simulink model "simulink_group46"  (R2022b)
settings: Solver=FixedStepAuto  StartTime=0.0  StopTime=10  FixedStep=1e-3  RelTol=1e-3  EnableMultiTasking=on
undefined symbols (not defined in the file): A0, A1, D0, D1, D10, D11, D12, D13, D2, D3, D4, D5, D6, D7, D8, D9, PTA0, PTA1, PTA2, PTB2, PTB23, PTB3, PTB9, PTC16, PTC17, PTC2, PTC3, PTC4, PTD0, PTD1, PTD2, PTD3
libraries: frdmk64flib x20, etargetslib x18, simulink x2, dspstat3 x1
(part 2 of 2)

== stateflow chart simulink_group46/Requirements Table ==
  (default) -> (junction 1073756783)
  (junction 1073756783) -> (junction 1073756784) : {
      | % SF_REQ_REV_07
      | }
  (junction 1073756784) -> (junction 1073756786) : {
      | % HEADER_ASSIGNMENTS
      |
      | }
  (junction 1073756786) -> (junction 1073756788) : {
      | % START_A_4
      | }
  (junction 1073756788) -> (junction 1073756790) : {
      | }
  (junction 1073756790) -> (junction 1073756792) : {
      | reqtable_assumption((LRL <= 175 && LRL >= 30 && LRL <= URL), 4);
      | }
  (junction 1073756792) -> (junction 1073756794) : {
      | }
  (junction 1073756794) -> (junction 1073756796) : {
      | % END_A_4
      | }
  (junction 1073756796) -> (junction 1073756798) : {
      | % START_A_7
      | }
  (junction 1073756798) -> (junction 1073756800) : {
      | }
  (junction 1073756800) -> (junction 1073756802) : {
      | reqtable_assumption((URL <= 175 && URL >= 50), 7);
      | }
  (junction 1073756802) -> (junction 1073756804) : {
      | }
  (junction 1073756804) -> (junction 1073756806) : {
      | % END_A_7
      | }
  (junction 1073756806) -> (junction 1073756808) : {
      | % START_A_10
      | }
  (junction 1073756808) -> (junction 1073756810) : {
      | }
  (junction 1073756810) -> (junction 1073756812) : {
      | reqtable_assumption((PACING_REF_PWM <= 64), 10);
      | }
  (junction 1073756812) -> (junction 1073756814) : {
      | }
  (junction 1073756814) -> (junction 1073756816) : {
      | % END_A_10
      | }
  (junction 1073756816) -> (junction 1073756818) : {
      | % START_A_16
      | }
  (junction 1073756818) -> (junction 1073756820) : {
      | }
  (junction 1073756820) -> (junction 1073756822) : {
      | reqtable_assumption((VRP >= 150 && VRP <= 500), 16);
      | }
  (junction 1073756822) -> (junction 1073756824) : {
      | }
  (junction 1073756824) -> (junction 1073756826) : {
      | % END_A_16
      | }
  (junction 1073756826) -> (junction 1073756828) : {
      | % START_A_19
      | }
  (junction 1073756828) -> (junction 1073756830) : {
      | }
  (junction 1073756830) -> (junction 1073756832) : {
      | reqtable_assumption((ARP >= 150 && ARP <= 500), 19);
      | }
  (junction 1073756832) -> (junction 1073756834) : {
      | }
  (junction 1073756834) -> (junction 1073756836) : {
      | % END_A_19
      | }
  (junction 1073756836) -> (junction 1073756838) : {
      | % START_A_22
      | }
  (junction 1073756838) -> (junction 1073756840) : {
      | }
  (junction 1073756840) -> (junction 1073756842) : {
      | reqtable_assumption((mode >= 0 && mode <= 8), 22);
      | }
  (junction 1073756842) -> (junction 1073756844) : {
      | }
  (junction 1073756844) -> (junction 1073756846) : {
      | % END_A_22
      | }
  (junction 1073756846) -> (junction 1073756848) : {
      | % START_R_1
      | }
  (junction 1073756848) -> (junction 1073756850) : {
      | }
  (junction 1073756850) -> (junction 1073756852)
  (junction 1073756852) -> (junction 1073756854) [order 1] : [(((mode) == (2))) && (((FRONTEND_CTRL) == (true))) && (((PACE_CHARGE_CTRL) == (true))) && (((PACE_GND_CTRL) == (true))) && (((ATR_CMP_DETECT) == (true)) || ((ATR_CMP_DETECT) == (false)))]
  (junction 1073756852) -> (junction 1073756896) [order 2]
  (junction 1073756854) -> (junction 1073756856) : {
      | reqtable_postcondition((((ATR_PACE_CTRL) == (false))) && (((ATR_GND_CTRL) == (true)) || ((ATR_GND_CTRL) == (false))), 'R:1');
      |
      |
      | }
  (junction 1073756856) -> (junction 1073756858) : {
      | }
  (junction 1073756858) -> (junction 1073756860) : {
      | % START_R_79
      | }
  (junction 1073756860) -> (junction 1073756862) : {
      | }
  (junction 1073756862) -> (junction 1073756864)
  (junction 1073756864) -> (junction 1073756866) [order 1] : [(((VENT_CMP_DETECT) == (false))) && (((prev_state) == (2)))]
  (junction 1073756864) -> (junction 1073756872) [order 2]
  (junction 1073756866) -> (junction 1073756868) : {
      | reqtable_postcondition((((VENT_PACE_CTRL) == (true))) && (((VENT_GND_CTRL) == (true))) && (((state) == (3))), 'R:1.1');
      |
      |
      | }
  (junction 1073756868) -> (junction 1073756870) : {
      | }
  (junction 1073756870) -> (junction 1073756872)
  (junction 1073756872) -> (junction 1073756874)
  (junction 1073756874) -> (junction 1073756876) : {
      | % END_R_79
      | }
  (junction 1073756876) -> (junction 1073756878) : {
      | % START_R_82
      | }
  (junction 1073756878) -> (junction 1073756880) : {
      | }
  (junction 1073756880) -> (junction 1073756882)
  (junction 1073756882) -> (junction 1073756884) [order 1] : [(((VENT_CMP_DETECT) == (true))) && (((prev_state) == (1)))]
  (junction 1073756882) -> (junction 1073756890) [order 2]
  (junction 1073756884) -> (junction 1073756886) : {
      | reqtable_postcondition((((VENT_PACE_CTRL) == (false))) && (((VENT_GND_CTRL) == (false))) && (((state) == (1))), 'R:1.2');
      |
      |
      | }
  (junction 1073756886) -> (junction 1073756888) : {
      | }
  (junction 1073756888) -> (junction 1073756890)
  (junction 1073756890) -> (junction 1073756892)
  (junction 1073756892) -> (junction 1073756894) : {
      | % END_R_82
      | }
  (junction 1073756894) -> (junction 1073756896)
  (junction 1073756896) -> (junction 1073756898)
  (junction 1073756898) -> (junction 1073756900) : {
      | % END_R_1
      | }
  (junction 1073756900) -> (junction 1073756902) : {
      | % START_R_28
      | }
  (junction 1073756902) -> (junction 1073756904) : {
      | }
  (junction 1073756904) -> (junction 1073756906)
  (junction 1073756906) -> (junction 1073756908) [order 1] : [(((mode) == (1)) || ((mode) == (2))) && (((FRONTEND_CTRL) == (false))) && (((PACE_CHARGE_CTRL) == (false))) && (((PACE_GND_CTRL) == (true))) && (((VENT_CMP_DETECT) == (false))) && (((ATR_CMP_DETECT) == (true)) || ((ATR_CMP_DETECT) == (false))) && (((prev_state) == (1)))]
  (junction 1073756906) -> (junction 1073756914) [order 2]
  (junction 1073756908) -> (junction 1073756910) : {
      | reqtable_postcondition((((VENT_PACE_CTRL) == (true))) && (((ATR_PACE_CTRL) == (false))) && (((VENT_GND_CTRL) == (false))) && (((ATR_GND_CTRL) == (true)) || ((ATR_GND_CTRL) == (false))) && (((state) == (1))), 'R:2');
      |
      |
      | }
  (junction 1073756910) -> (junction 1073756912) : {
      | }
  (junction 1073756912) -> (junction 1073756914)
  (junction 1073756914) -> (junction 1073756916)
  (junction 1073756916) -> (junction 1073756918) : {
      | % END_R_28
      | }
  (junction 1073756918) -> (junction 1073756920) : {
      | % START_R_46
      | }
  (junction 1073756920) -> (junction 1073756922) : {
      | }
  (junction 1073756922) -> (junction 1073756924) : {
      |
      |
      | }
  (junction 1073756924) -> (junction 1073756926) : {
      | }
  (junction 1073756926) -> (junction 1073756928) : {
      | % START_R_61
      | }
  (junction 1073756928) -> (junction 1073756930) : {
      | }
  (junction 1073756930) -> (junction 1073756932)
  (junction 1073756932) -> (junction 1073756934) [order 1] : [(((mode) == (1))) && (((FRONTEND_CTRL) == (false))) && (((PACE_CHARGE_CTRL) == (true))) && (((PACE_GND_CTRL) == (true))) && (((VENT_CMP_DETECT) == (true)) || ((VENT_CMP_DETECT) == (false))) && (((ATR_CMP_DETECT) == (true)) || ((ATR_CMP_DETECT) == (false))) && (((prev_state) == (2)))]
  (junction 1073756932) -> (junction 1073756940) [order 2]
  (junction 1073756934) -> (junction 1073756936) : {
      | reqtable_postcondition((((VENT_PACE_CTRL) == (false))) && (((ATR_PACE_CTRL) == (true)) || ((ATR_PACE_CTRL) == (false))) && (((VENT_GND_CTRL) == (true))) && (((ATR_GND_CTRL) == (true)) || ((ATR_GND_CTRL) == (false))) && (((state) == (2))), 'R:3.1');
      |
      |
      | }
  (junction 1073756936) -> (junction 1073756938) : {
      | }
  (junction 1073756938) -> (junction 1073756940)
  (junction 1073756940) -> (junction 1073756942)
  (junction 1073756942) -> (junction 1073756944) : {
      | % END_R_61
      | }
  (junction 1073756944) -> (junction 1073756946) : {
      | % START_R_64
      | }
  (junction 1073756946) -> (junction 1073756948) : {
      | }
  (junction 1073756948) -> (junction 1073756950)
  (junction 1073756950) -> (junction 1073756952) [order 1] : [(((mode) == (2))) && (((FRONTEND_CTRL) == (true)) || ((FRONTEND_CTRL) == (false))) && (((PACE_CHARGE_CTRL) == (true))) && (((PACE_GND_CTRL) == (true))) && (((VENT_CMP_DETECT) == (true)) || ((VENT_CMP_DETECT) == (false))) && (((ATR_CMP_DETECT) == (true)) || ((ATR_CMP_DETECT) == (false))) && (((prev_state) == (1)))]
  (junction 1073756950) -> (junction 1073756958) [order 2]
  (junction 1073756952) -> (junction 1073756954) : {
      | reqtable_postcondition((((VENT_PACE_CTRL) == (false))) && (((ATR_PACE_CTRL) == (true)) || ((ATR_PACE_CTRL) == (false))) && (((VENT_GND_CTRL) == (true))) && (((ATR_GND_CTRL) == (true)) || ((ATR_GND_CTRL) == (false))) && (((state) == (2))), 'R:3.2');
      |
      |
      | }
  (junction 1073756954) -> (junction 1073756956) : {
      | }
  (junction 1073756956) -> (junction 1073756958)
  (junction 1073756958) -> (junction 1073756960)
  (junction 1073756960) -> (junction 1073756962) : {
      | % END_R_64
      | }
  (junction 1073756962) -> (junction 1073756964) : {
      | % END_R_46
      | }
  (junction 1073756964) -> (junction 1073756966) : {
      | % START_R_31
      | }
  (junction 1073756966) -> (junction 1073756968) : {
      | }
  (junction 1073756968) -> (junction 1073756970)
  (junction 1073756970) -> (junction 1073756972) [order 1] : [(((mode) == (4))) && (((FRONTEND_CTRL) == (true))) && (((PACE_CHARGE_CTRL) == (true))) && (((PACE_GND_CTRL) == (true))) && (((VENT_CMP_DETECT) == (true)) || ((VENT_CMP_DETECT) == (false)))]
  (junction 1073756970) -> (junction 1073757014) [order 2]
  (junction 1073756972) -> (junction 1073756974) : {
      | reqtable_postcondition((((VENT_PACE_CTRL) == (false))) && (((VENT_GND_CTRL) == (true)) || ((VENT_GND_CTRL) == (false))), 'R:4');
      |
      |
      | }
  (junction 1073756974) -> (junction 1073756976) : {
      | }
  (junction 1073756976) -> (junction 1073756978) : {
      | % START_R_85
      | }
  (junction 1073756978) -> (junction 1073756980) : {
      | }
  (junction 1073756980) -> (junction 1073756982)
  (junction 1073756982) -> (junction 1073756984) [order 1] : [(((ATR_CMP_DETECT) == (false))) && (((prev_state) == (2)))]
  (junction 1073756982) -> (junction 1073756990) [order 2]
  (junction 1073756984) -> (junction 1073756986) : {
      | reqtable_postcondition((((ATR_PACE_CTRL) == (true))) && (((ATR_GND_CTRL) == (true))) && (((state) == (3))), 'R:4.1');
      |
      |
      | }
  (junction 1073756986) -> (junction 1073756988) : {
      | }
  (junction 1073756988) -> (junction 1073756990)
  (junction 1073756990) -> (junction 1073756992)
  (junction 1073756992) -> (junction 1073756994) : {
      | % END_R_85
      | }
  (junction 1073756994) -> (junction 1073756996) : {
      | % START_R_88
      | }
  (junction 1073756996) -> (junction 1073756998) : {
      | }
  (junction 1073756998) -> (junction 1073757000)
  (junction 1073757000) -> (junction 1073757002) [order 1] : [(((ATR_CMP_DETECT) == (true))) && (((prev_state) == (1)))]
  (junction 1073757000) -> (junction 1073757008) [order 2]
  (junction 1073757002) -> (junction 1073757004) : {
      | reqtable_postcondition((((ATR_PACE_CTRL) == (false))) && (((ATR_GND_CTRL) == (false))) && (((state) == (1))), 'R:4.2');
      |
      |
      | }
  (junction 1073757004) -> (junction 1073757006) : {
      | }
  (junction 1073757006) -> (junction 1073757008)
  (junction 1073757008) -> (junction 1073757010)
  (junction 1073757010) -> (junction 1073757012) : {
      | % END_R_88
      | }
  (junction 1073757012) -> (junction 1073757014)
  (junction 1073757014) -> (junction 1073757016)
  (junction 1073757016) -> (junction 1073757018) : {
      | % END_R_31
      | }
  (junction 1073757018) -> (junction 1073757020) : {
      | % START_R_37
      | }
  (junction 1073757020) -> (junction 1073757022) : {
      | }
  (junction 1073757022) -> (junction 1073757024)
  (junction 1073757024) -> (junction 1073757026) [order 1] : [(((mode) == (3)) || ((mode) == (4))) && (((FRONTEND_CTRL) == (false))) && (((PACE_CHARGE_CTRL) == (false))) && (((PACE_GND_CTRL) == (true))) && (((VENT_CMP_DETECT) == (true)) || ((VENT_CMP_DETECT) == (false))) && (((ATR_CMP_DETECT) == (false))) && (((prev_state) == (1)))]
  (junction 1073757024) -> (junction 1073757032) [order 2]
  (junction 1073757026) -> (junction 1073757028) : {
      | reqtable_postcondition((((VENT_PACE_CTRL) == (false))) && (((ATR_PACE_CTRL) == (true))) && (((VENT_GND_CTRL) == (true)) || ((VENT_GND_CTRL) == (false))) && (((ATR_GND_CTRL) == (false))) && (((state) == (1))), 'R:5');
      |
      |
      | }
  (junction 1073757028) -> (junction 1073757030) : {
      | }
  (junction 1073757030) -> (junction 1073757032)
  (junction 1073757032) -> (junction 1073757034)
  (junction 1073757034) -> (junction 1073757036) : {
      | % END_R_37
      | }
  (junction 1073757036) -> (junction 1073757038) : {
      | % START_R_55
      | }
  (junction 1073757038) -> (junction 1073757040) : {
      | }
  (junction 1073757040) -> (junction 1073757042) : {
      |
      |
      | }
  (junction 1073757042) -> (junction 1073757044) : {
      | }
  (junction 1073757044) -> (junction 1073757046) : {
      | % START_R_67
      | }
  (junction 1073757046) -> (junction 1073757048) : {
      | }
  (junction 1073757048) -> (junction 1073757050)
  (junction 1073757050) -> (junction 1073757052) [order 1] : [(((mode) == (3))) && (((FRONTEND_CTRL) == (false))) && (((PACE_CHARGE_CTRL) == (true))) && (((PACE_GND_CTRL) == (true))) && (((VENT_CMP_DETECT) == (true)) || ((VENT_CMP_DETECT) == (false))) && (((ATR_CMP_DETECT) == (true)) || ((ATR_CMP_DETECT) == (false))) && (((prev_state) == (2)))]
  (junction 1073757050) -> (junction 1073757058) [order 2]
  (junction 1073757052) -> (junction 1073757054) : {
      | reqtable_postcondition((((VENT_PACE_CTRL) == (true)) || ((VENT_PACE_CTRL) == (false))) && (((ATR_PACE_CTRL) == (false))) && (((VENT_GND_CTRL) == (true)) || ((VENT_GND_CTRL) == (false))) && (((ATR_GND_CTRL) == (true))) && (((state) == (2))), 'R:6.1');
      |
      |
      | }
  (junction 1073757054) -> (junction 1073757056) : {
      | }
  (junction 1073757056) -> (junction 1073757058)
  (junction 1073757058) -> (junction 1073757060)
  (junction 1073757060) -> (junction 1073757062) : {
      | % END_R_67
      | }
  (junction 1073757062) -> (junction 1073757064) : {
      | % START_R_70
      | }
  (junction 1073757064) -> (junction 1073757066) : {
      | }
  (junction 1073757066) -> (junction 1073757068)
  (junction 1073757068) -> (junction 1073757070) [order 1] : [(((mode) == (4))) && (((FRONTEND_CTRL) == (true)) || ((FRONTEND_CTRL) == (false))) && (((PACE_CHARGE_CTRL) == (true))) && (((PACE_GND_CTRL) == (true))) && (((VENT_CMP_DETECT) == (true)) || ((VENT_CMP_DETECT) == (false))) && (((ATR_CMP_DETECT) == (true)) || ((ATR_CMP_DETECT) == (false))) && (((prev_state) == (1)))]
  (junction 1073757068) -> (junction 1073757076) [order 2]
  (junction 1073757070) -> (junction 1073757072) : {
      | reqtable_postcondition((((VENT_PACE_CTRL) == (true)) || ((VENT_PACE_CTRL) == (false))) && (((ATR_PACE_CTRL) == (false))) && (((VENT_GND_CTRL) == (true)) || ((VENT_GND_CTRL) == (false))) && (((ATR_GND_CTRL) == (true))) && (((state) == (2))), 'R:6.2');
      |
      |
      | }
  (junction 1073757072) -> (junction 1073757074) : {
      | }
  (junction 1073757074) -> (junction 1073757076)
  (junction 1073757076) -> (junction 1073757078)
  (junction 1073757078) -> (junction 1073757080) : {
      | % END_R_70
      | }
  (junction 1073757080) -> (junction 1073757082) : {
      | % END_R_55
      | }
  (junction 1073757082) -> (junction 1073757084) : {
      | % START_R_91
      | }
  (junction 1073757084) -> (junction 1073757086) : {
      | }
  (junction 1073757086) -> (junction 1073757088)
  (junction 1073757088) -> (junction 1073757090) [order 1] : [(((mode) == (6))) && (((FRONTEND_CTRL) == (true))) && (((PACE_CHARGE_CTRL) == (true))) && (((PACE_GND_CTRL) == (true))) && (((ATR_CMP_DETECT) == (true)) || ((ATR_CMP_DETECT) == (false)))]
  (junction 1073757088) -> (junction 1073757132) [order 2]
  (junction 1073757090) -> (junction 1073757092) : {
      | reqtable_postcondition((((ATR_PACE_CTRL) == (false))) && (((ATR_GND_CTRL) == (true)) || ((ATR_GND_CTRL) == (false))), 'R:7');
      |
      |
      | }
  (junction 1073757092) -> (junction 1073757094) : {
      | }
  (junction 1073757094) -> (junction 1073757096) : {
      | % START_R_94
      | }
  (junction 1073757096) -> (junction 1073757098) : {
      | }
  (junction 1073757098) -> (junction 1073757100)
  (junction 1073757100) -> (junction 1073757102) [order 1] : [(((VENT_CMP_DETECT) == (false))) && (((prev_state) == (2)))]
  (junction 1073757100) -> (junction 1073757108) [order 2]
  (junction 1073757102) -> (junction 1073757104) : {
      | reqtable_postcondition((((VENT_PACE_CTRL) == (true))) && (((VENT_GND_CTRL) == (true))) && (((state) == (3))), 'R:7.1');
      |
      |
      | }
  (junction 1073757104) -> (junction 1073757106) : {
      | }
  (junction 1073757106) -> (junction 1073757108)
  (junction 1073757108) -> (junction 1073757110)
  (junction 1073757110) -> (junction 1073757112) : {
      | % END_R_94
      | }
  (junction 1073757112) -> (junction 1073757114) : {
      | % START_R_97
      | }
  (junction 1073757114) -> (junction 1073757116) : {
      | }
  (junction 1073757116) -> (junction 1073757118)
  (junction 1073757118) -> (junction 1073757120) [order 1] : [(((VENT_CMP_DETECT) == (true))) && (((prev_state) == (1)))]
  (junction 1073757118) -> (junction 1073757126) [order 2]
  (junction 1073757120) -> (junction 1073757122) : {
      | reqtable_postcondition((((VENT_PACE_CTRL) == (false))) && (((VENT_GND_CTRL) == (false))) && (((state) == (1))), 'R:7.2');
      |
      |
      | }
  (junction 1073757122) -> (junction 1073757124) : {
      | }
  (junction 1073757124) -> (junction 1073757126)
  (junction 1073757126) -> (junction 1073757128)
  (junction 1073757128) -> (junction 1073757130) : {
      | % END_R_97
      | }
  (junction 1073757130) -> (junction 1073757132)
  (junction 1073757132) -> (junction 1073757134)
  (junction 1073757134) -> (junction 1073757136) : {
      | % END_R_91
      | }
  (junction 1073757136) -> (junction 1073757138) : {
      | % START_R_100
      | }
  (junction 1073757138) -> (junction 1073757140) : {
      | }
  (junction 1073757140) -> (junction 1073757142)
  (junction 1073757142) -> (junction 1073757144) [order 1] : [(((mode) == (5)) || ((mode) == (6))) && (((FRONTEND_CTRL) == (false))) && (((PACE_CHARGE_CTRL) == (false))) && (((PACE_GND_CTRL) == (true))) && (((VENT_CMP_DETECT) == (false))) && (((ATR_CMP_DETECT) == (true)) || ((ATR_CMP_DETECT) == (false))) && (((prev_state) == (1)))]
  (junction 1073757142) -> (junction 1073757150) [order 2]
  (junction 1073757144) -> (junction 1073757146) : {
      | reqtable_postcondition((((VENT_PACE_CTRL) == (true))) && (((ATR_PACE_CTRL) == (false))) && (((VENT_GND_CTRL) == (false))) && (((ATR_GND_CTRL) == (true)) || ((ATR_GND_CTRL) == (false))) && (((state) == (1))), 'R:8');
      |
      |
      | }
  (junction 1073757146) -> (junction 1073757148) : {
      | }
  (junction 1073757148) -> (junction 1073757150)
  (junction 1073757150) -> (junction 1073757152)
  (junction 1073757152) -> (junction 1073757154) : {
      | % END_R_100
      | }
  (junction 1073757154) -> (junction 1073757156) : {
      | % START_R_103
      | }
  (junction 1073757156) -> (junction 1073757158) : {
      | }
  (junction 1073757158) -> (junction 1073757160) : {
      |
      |
      | }
  (junction 1073757160) -> (junction 1073757162) : {
      | }
  (junction 1073757162) -> (junction 1073757164) : {
      | % START_R_106
      | }
  (junction 1073757164) -> (junction 1073757166) : {
      | }
  (junction 1073757166) -> (junction 1073757168)
  (junction 1073757168) -> (junction 1073757170) [order 1] : [(((mode) == (5))) && (((FRONTEND_CTRL) == (false))) && (((PACE_CHARGE_CTRL) == (true))) && (((PACE_GND_CTRL) == (true))) && (((VENT_CMP_DETECT) == (true)) || ((VENT_CMP_DETECT) == (false))) && (((ATR_CMP_DETECT) == (true)) || ((ATR_CMP_DETECT) == (false))) && (((prev_state) == (2)))]
  (junction 1073757168) -> (junction 1073757176) [order 2]
  (junction 1073757170) -> (junction 1073757172) : {
      | reqtable_postcondition((((VENT_PACE_CTRL) == (false))) && (((ATR_PACE_CTRL) == (true)) || ((ATR_PACE_CTRL) == (false))) && (((VENT_GND_CTRL) == (true))) && (((ATR_GND_CTRL) == (true)) || ((ATR_GND_CTRL) == (false))) && (((state) == (2))), 'R:9.1');
      |
      |
      | }
  (junction 1073757172) -> (junction 1073757174) : {
      | }
  (junction 1073757174) -> (junction 1073757176)
  (junction 1073757176) -> (junction 1073757178)
  (junction 1073757178) -> (junction 1073757180) : {
      | % END_R_106
      | }
  (junction 1073757180) -> (junction 1073757182) : {
      | % START_R_109
      | }
  (junction 1073757182) -> (junction 1073757184) : {
      | }
  (junction 1073757184) -> (junction 1073757186)
  (junction 1073757186) -> (junction 1073757188) [order 1] : [(((mode) == (6))) && (((FRONTEND_CTRL) == (true)) || ((FRONTEND_CTRL) == (false))) && (((PACE_CHARGE_CTRL) == (true))) && (((PACE_GND_CTRL) == (true))) && (((VENT_CMP_DETECT) == (true)) || ((VENT_CMP_DETECT) == (false))) && (((ATR_CMP_DETECT) == (true)) || ((ATR_CMP_DETECT) == (false))) && (((prev_state) == (1)))]
  (junction 1073757186) -> (junction 1073757194) [order 2]
  (junction 1073757188) -> (junction 1073757190) : {
      | reqtable_postcondition((((VENT_PACE_CTRL) == (false))) && (((ATR_PACE_CTRL) == (true)) || ((ATR_PACE_CTRL) == (false))) && (((VENT_GND_CTRL) == (true))) && (((ATR_GND_CTRL) == (true)) || ((ATR_GND_CTRL) == (false))) && (((state) == (2))), 'R:9.2');
      |
      |
      | }
  (junction 1073757190) -> (junction 1073757192) : {
      | }
  (junction 1073757192) -> (junction 1073757194)
  (junction 1073757194) -> (junction 1073757196)
  (junction 1073757196) -> (junction 1073757198) : {
      | % END_R_109
      | }
  (junction 1073757198) -> (junction 1073757200) : {
      | % END_R_103
      | }
  (junction 1073757200) -> (junction 1073757202) : {
      | % START_R_112
      | }
  (junction 1073757202) -> (junction 1073757204) : {
      | }
  (junction 1073757204) -> (junction 1073757206)
  (junction 1073757206) -> (junction 1073757208) [order 1] : [(((mode) == (8))) && (((FRONTEND_CTRL) == (true))) && (((PACE_CHARGE_CTRL) == (true))) && (((PACE_GND_CTRL) == (true))) && (((VENT_CMP_DETECT) == (true)) || ((VENT_CMP_DETECT) == (false)))]
  (junction 1073757206) -> (junction 1073757250) [order 2]
  (junction 1073757208) -> (junction 1073757210) : {
      | reqtable_postcondition((((VENT_PACE_CTRL) == (false))) && (((VENT_GND_CTRL) == (true)) || ((VENT_GND_CTRL) == (false))), 'R:10');
      |
      |
      | }
  (junction 1073757210) -> (junction 1073757212) : {
      | }
  (junction 1073757212) -> (junction 1073757214) : {
      | % START_R_115
      | }
  (junction 1073757214) -> (junction 1073757216) : {
      | }
  (junction 1073757216) -> (junction 1073757218)
  (junction 1073757218) -> (junction 1073757220) [order 1] : [(((ATR_CMP_DETECT) == (false))) && (((prev_state) == (2)))]
  (junction 1073757218) -> (junction 1073757226) [order 2]
  (junction 1073757220) -> (junction 1073757222) : {
      | reqtable_postcondition((((ATR_PACE_CTRL) == (true))) && (((ATR_GND_CTRL) == (true))) && (((state) == (3))), 'R:10.1');
      |
      |
      | }
  (junction 1073757222) -> (junction 1073757224) : {
      | }
  (junction 1073757224) -> (junction 1073757226)
  (junction 1073757226) -> (junction 1073757228)
  (junction 1073757228) -> (junction 1073757230) : {
      | % END_R_115
      | }
  (junction 1073757230) -> (junction 1073757232) : {
      | % START_R_118
      | }
  (junction 1073757232) -> (junction 1073757234) : {
      | }
  (junction 1073757234) -> (junction 1073757236)
  (junction 1073757236) -> (junction 1073757238) [order 1] : [(((ATR_CMP_DETECT) == (true))) && (((prev_state) == (1)))]
  (junction 1073757236) -> (junction 1073757244) [order 2]
  (junction 1073757238) -> (junction 1073757240) : {
      | reqtable_postcondition((((ATR_PACE_CTRL) == (false))) && (((ATR_GND_CTRL) == (false))) && (((state) == (1))), 'R:10.2');
      |
      |
      | }
  (junction 1073757240) -> (junction 1073757242) : {
      | }
  (junction 1073757242) -> (junction 1073757244)
  (junction 1073757244) -> (junction 1073757246)
  (junction 1073757246) -> (junction 1073757248) : {
      | % END_R_118
      | }
  (junction 1073757248) -> (junction 1073757250)
  (junction 1073757250) -> (junction 1073757252)
  (junction 1073757252) -> (junction 1073757254) : {
      | % END_R_112
      | }
  (junction 1073757254) -> (junction 1073757256) : {
      | % START_R_121
      | }
  (junction 1073757256) -> (junction 1073757258) : {
      | }
  (junction 1073757258) -> (junction 1073757260)
  (junction 1073757260) -> (junction 1073757262) [order 1] : [(((mode) == (7)) || ((mode) == (8))) && (((FRONTEND_CTRL) == (false))) && (((PACE_CHARGE_CTRL) == (false))) && (((PACE_GND_CTRL) == (true))) && (((VENT_CMP_DETECT) == (true)) || ((VENT_CMP_DETECT) == (false))) && (((ATR_CMP_DETECT) == (false))) && (((prev_state) == (1)))]
  (junction 1073757260) -> (junction 1073757268) [order 2]
  (junction 1073757262) -> (junction 1073757264) : {
      | reqtable_postcondition((((VENT_PACE_CTRL) == (false))) && (((ATR_PACE_CTRL) == (true))) && (((VENT_GND_CTRL) == (true)) || ((VENT_GND_CTRL) == (false))) && (((ATR_GND_CTRL) == (false))) && (((state) == (1))), 'R:11');
      |
      |
      | }
  (junction 1073757264) -> (junction 1073757266) : {
      | }
  (junction 1073757266) -> (junction 1073757268)
  (junction 1073757268) -> (junction 1073757270)
  (junction 1073757270) -> (junction 1073757272) : {
      | % END_R_121
      | }
  (junction 1073757272) -> (junction 1073757274) : {
      | % START_R_124
      | }
  (junction 1073757274) -> (junction 1073757276) : {
      | }
  (junction 1073757276) -> (junction 1073757278) : {
      |
      |
      | }
  (junction 1073757278) -> (junction 1073757280) : {
      | }
  (junction 1073757280) -> (junction 1073757282) : {
      | % START_R_127
      | }
  (junction 1073757282) -> (junction 1073757284) : {
      | }
  (junction 1073757284) -> (junction 1073757286)
  (junction 1073757286) -> (junction 1073757288) [order 1] : [(((mode) == (7))) && (((FRONTEND_CTRL) == (false))) && (((PACE_CHARGE_CTRL) == (true))) && (((PACE_GND_CTRL) == (true))) && (((VENT_CMP_DETECT) == (true)) || ((VENT_CMP_DETECT) == (false))) && (((ATR_CMP_DETECT) == (true)) || ((ATR_CMP_DETECT) == (false))) && (((prev_state) == (2)))]
  (junction 1073757286) -> (junction 1073757294) [order 2]
  (junction 1073757288) -> (junction 1073757290) : {
      | reqtable_postcondition((((VENT_PACE_CTRL) == (true)) || ((VENT_PACE_CTRL) == (false))) && (((ATR_PACE_CTRL) == (false))) && (((VENT_GND_CTRL) == (true)) || ((VENT_GND_CTRL) == (false))) && (((ATR_GND_CTRL) == (true))) && (((state) == (2))), 'R:12.1');
      |
      |
      | }
  (junction 1073757290) -> (junction 1073757292) : {
      | }
  (junction 1073757292) -> (junction 1073757294)
  (junction 1073757294) -> (junction 1073757296)
  (junction 1073757296) -> (junction 1073757298) : {
      | % END_R_127
      | }
  (junction 1073757298) -> (junction 1073757300) : {
      | % START_R_130
      | }
  (junction 1073757300) -> (junction 1073757302) : {
      | }
  (junction 1073757302) -> (junction 1073757304)
  (junction 1073757304) -> (junction 1073757306) [order 1] : [(((mode) == (8))) && (((FRONTEND_CTRL) == (true)) || ((FRONTEND_CTRL) == (false))) && (((PACE_CHARGE_CTRL) == (true))) && (((PACE_GND_CTRL) == (true))) && (((VENT_CMP_DETECT) == (true)) || ((VENT_CMP_DETECT) == (false))) && (((ATR_CMP_DETECT) == (true)) || ((ATR_CMP_DETECT) == (false))) && (((prev_state) == (1)))]
  (junction 1073757304) -> (junction 1073757312) [order 2]
  (junction 1073757306) -> (junction 1073757308) : {
      | reqtable_postcondition((((VENT_PACE_CTRL) == (true)) || ((VENT_PACE_CTRL) == (false))) && (((ATR_PACE_CTRL) == (false))) && (((VENT_GND_CTRL) == (true)) || ((VENT_GND_CTRL) == (false))) && (((ATR_GND_CTRL) == (true))) && (((state) == (2))), 'R:12.2');
      |
      |
      | }
  (junction 1073757308) -> (junction 1073757310) : {
      | }
  (junction 1073757310) -> (junction 1073757312)
  (junction 1073757312) -> (junction 1073757314)
  (junction 1073757314) -> (junction 1073757316) : {
      | % END_R_130
      | }
  (junction 1073757316) -> (junction 1073757414) : {
      | % END_R_124
      | }
  (junction 1073757414) -> (junction 1073757416) : {
      | % START_R_76
      | }
  (junction 1073757416) -> (junction 1073757418) : {
      | }
  (junction 1073757418) -> (junction 1073757420)
  (junction 1073757420) -> (junction 1073757422) [order 1] : [(((mode) == (0)) || ((mode) == (1)) || ((mode) == (2)) || ((mode) == (3)) || ((mode) == (4)) || ((mode) == (5)) || ((mode) == (6)) || ((mode) == (7)) || ((mode) == (8))) && (((prev_state) >= (0) && (prev_state) <= (3)))]
  (junction 1073757420) -> (junction 1073757428) [order 2]
  (junction 1073757422) -> (junction 1073757424) : {
      | reqtable_postcondition((((VENT_PACE_CTRL) == (true)) || ((VENT_PACE_CTRL) == (false))) && (((ATR_PACE_CTRL) == (true)) || ((ATR_PACE_CTRL) == (false))) && (((VENT_GND_CTRL) == (true)) || ((VENT_GND_CTRL) == (false))) && (((ATR_GND_CTRL) == (true)) || ((ATR_GND_CTRL) == (false))) && (((state) >= (0) && (state) <= (3))), 'R:13');
      |
      |
      | }
  (junction 1073757424) -> (junction 1073757426) : {
      | }
  (junction 1073757426) -> (junction 1073757428)
  (junction 1073757428) -> (junction 1073757430)
  (junction 1073757430) -> (junction 1073757432) : {
      | % END_R_76
      | }
  data: LRL input; URL input double; ARP input double; VRP input double; mode input int16; VENT_CMP_DETECT input boolean; ATR_CMP_DETECT input boolean; PACING_REF_PWM input double; FRONTEND_CTRL input boolean; ATR_PACE_CTRL input boolean; VENT_PACE_CTRL input boolean; PACE_GND_CTRL input boolean; PACE_CHARGE_CTRL input boolean; ATR_GND_CTRL input boolean; VENT_GND_CTRL input boolean; state input int16; prev_state input int16

== stateflow chart simulink_group46/PACING MODES ==
  state VOO [group]
    state Charge_C22_VOO
      entry:
      %Charge C22
      ATR_PACE_CTRL = false;
      VENT_PACE_CTRL = false;
      PACING_REF_PWM = (VAmplitude/5)*100;
      PACE_CHARGE_CTRL = true;
      %Discharge C21
      PACE_GND_CTRL = true;
      VENT_PACE_CTRL = false;
      Z_ATR_CTRL = false;
      Z_VENT_CTRL = false;
      ATR_PACE_CTRL = false;
      ATR_GND_CTRL = false;
      VENT_GND_CTRL = true;
      state = 1;
      prev_state = 2;
    state Discharge_C22_VENT_VOO
      entry:
      %Disharge C22
      PACE_CHARGE_CTRL = false;
      PACE_GND_CTRL = true;
      ATR_PACE_CTRL = false;
      ATR_GND_CTRL = false;
      Z_ATR_CTRL = false;
      Z_VENT_CTRL = false;
      VENT_GND_CTRL = false;
      VENT_PACE_CTRL = true;
      state = 2;
      prev_state = 1;
    VOO.Discharge_C22_VENT_VOO -> VOO.Charge_C22_VOO : [after(LRI,msec)]
    VOO.Charge_C22_VOO -> VOO.Discharge_C22_VENT_VOO [order 2] : [after(VentWidth,msec)]
  state VOOR [group]
    state Charge_C22_VOO
      entry:
      %Charge C22
      ATR_PACE_CTRL = false;
      VENT_PACE_CTRL = false;
      PACING_REF_PWM = (VAmplitude/5)*100;
      PACE_CHARGE_CTRL = true;
      %Discharge C21
      PACE_GND_CTRL = true;
      VENT_PACE_CTRL = false;
      Z_ATR_CTRL = false;
      Z_VENT_CTRL = false;
      ATR_PACE_CTRL = false;
      ATR_GND_CTRL = false;
      VENT_GND_CTRL = true;
      state = 1;
      prev_state = 2;
    state Discharge_C22_VENT_VOO
      entry:
      %Discharge C22
      PACE_CHARGE_CTRL = false;
      PACE_GND_CTRL = true;
      ATR_PACE_CTRL = false;
      ATR_GND_CTRL = false;
      Z_ATR_CTRL = false;
      Z_VENT_CTRL = false;
      VENT_GND_CTRL = false;
      VENT_PACE_CTRL = true;
      state = 2;
      prev_state = 1;
    VOOR.Discharge_C22_VENT_VOO -> VOOR.Charge_C22_VOO : [after(interval,msec)]
    VOOR.Charge_C22_VOO -> VOOR.Discharge_C22_VENT_VOO : [after(VentWidth,msec)]
  state VVI [group]
    state Wait_VVI %(Refractory Period)
      entry:
      VENT_CMP_REF_PWM = (VentSensitivity/5)*100;
      FRONTEND_CTRL = true;
      %Discharge C21 and Charge C22
      PACE_GND_CTRL = true;
      VENT_PACE_CTRL = false;
      Z_ATR_CTRL = false;
      Z_VENT_CTRL = false;
      ATR_PACE_CTRL = false;
      ATR_GND_CTRL = false;
      VENT_GND_CTRL = true;
      PACING_REF_PWM = (VAmplitude/5)*100;
      PACE_CHARGE_CTRL = true;
      state = 1;
    state Sensing_Charge_C22_VVI %(Alert Period)
      entry:
      %Sensing turns on
      FRONTEND_CTRL = true;
      %Charge C22
      ATR_PACE_CTRL = false;
      VENT_PACE_CTRL = false;
      PACING_REF_PWM = (VAmplitude/5)*100;
      PACE_CHARGE_CTRL = true;
      state = 2;
      prev_state = 1;
    state Discharge_C22_VENT_VVI %(Pacing)
      entry:
      %Discharge C22, Sensing turns off
      FRONTEND_CTRL = false;
      PACE_CHARGE_CTRL = false;
      PACE_GND_CTRL = true;
      ATR_PACE_CTRL = false;
      ATR_GND_CTRL = false;
      Z_ATR_CTRL = false;
      Z_VENT_CTRL = false;
      VENT_GND_CTRL = false;
      VENT_PACE_CTRL = true;
      state = 3;
      prev_state = 2;
    VVI.Wait_VVI %(Refractory Period) -> VVI.Sensing_Charge_C22_VVI %(Alert Period) [order 2] : [after(VRP, msec)]
    VVI.Sensing_Charge_C22_VVI %(Alert Period) -> VVI.Wait_VVI %(Refractory Period) [order 1] : [VENT_CMP_DETECT == true]{natural = true}
    VVI.Wait_VVI %(Refractory Period) -> VVI.Wait_VVI %(Refractory Period) [order 3] : [VENT_CMP_DETECT == true]
    VVI.Sensing_Charge_C22_VVI %(Alert Period) -> VVI.Discharge_C22_VENT_VVI %(Pacing) [order 2] : [after(LRI-VRP,msec) & VENT_CMP_DETECT == false & natural == true]{natural = false}
    VVI.Sensing_Charge_C22_VVI %(Alert Period) -> VVI.Discharge_C22_VENT_VVI %(Pacing) [order 3] : [after(LRI-VRP-VentWidth,msec) & VENT_CMP_DETECT == false & natural == false]
    VVI.Discharge_C22_VENT_VVI %(Pacing) -> VVI.Wait_VVI %(Refractory Period) : [after(VentWidth,msec)]
  state VVIR [group]
    state Wait_VVI %(Refractory Period)
      entry:
      VENT_CMP_REF_PWM = (VentSensitivity/5)*100;
      FRONTEND_CTRL = false;
      %Discharge C21 and Charge C22
      PACE_GND_CTRL = true;
      VENT_PACE_CTRL = false;
      Z_ATR_CTRL = false;
      Z_VENT_CTRL = false;
      ATR_PACE_CTRL = false;
      ATR_GND_CTRL = false;
      VENT_GND_CTRL = true;
      PACING_REF_PWM = (VAmplitude/5)*100;
      PACE_CHARGE_CTRL = true;
      state = 1;
    state Sensing_Charge_C22_VVI %(Alert Period)
      entry:
      %Sensing turns on
      FRONTEND_CTRL = true;
      %Charge C22
      ATR_PACE_CTRL = false;
      VENT_PACE_CTRL = false;
      PACING_REF_PWM = (VAmplitude/5)*100;
      PACE_CHARGE_CTRL = true;
      state = 2;
      prev_state = 1;
    state Discharge_C22_VENT_VVI %(Pacing)
      entry:
      %Discharge C22, Sensing turns off
      PACE_CHARGE_CTRL = false;
      PACE_GND_CTRL = true;
      ATR_PACE_CTRL = false;
      ATR_GND_CTRL = false;
      Z_ATR_CTRL = false;
      Z_VENT_CTRL = false;
      VENT_GND_CTRL = false;
      VENT_PACE_CTRL = true;
      state = 3;
      prev_state = 2;
    VVIR.Wait_VVI %(Refractory Period) -> VVIR.Sensing_Charge_C22_VVI %(Alert Period) : [after(VRP, msec)]
    VVIR.Sensing_Charge_C22_VVI %(Alert Period) -> VVIR.Wait_VVI %(Refractory Period) [order 1] : [VENT_CMP_DETECT == true]{natural = true}
    VVIR.Sensing_Charge_C22_VVI %(Alert Period) -> VVIR.Discharge_C22_VENT_VVI %(Pacing) [order 3] : [after(interval-VRP-VentWidth,msec) & VENT_CMP_DETECT == false & natural == false]
    VVIR.Sensing_Charge_C22_VVI %(Alert Period) -> VVIR.Discharge_C22_VENT_VVI %(Pacing) [order 2] : [after(interval-VRP,msec) & VENT_CMP_DETECT == false & natural == true]{natural = false}
    VVIR.Discharge_C22_VENT_VVI %(Pacing) -> VVIR.Wait_VVI %(Refractory Period) : [after(VentWidth,msec)]
  state Mode_Selector
    %Determines the mode from the 8 listed below
    entry:
    state = 0;
    prev_state = 0;
    natural = false;
    LRI = 60000/LRL;
    interval=60000/AdaptiveRate;
    %Mode 1: VOO
    %Mode 2: VVI
    %Mode 3: AOO
    %Mode 4: AAI
    %Mode 5: VOOR
    %Mode 6: VVIR
    %Mode 7: AOOR
    %Mode 8: AAIR
  state AOO [group]
    state Charge_C22_AOO
      entry:
      %Charge C22
      ATR_PACE_CTRL = false;
      VENT_PACE_CTRL = false;
      PACING_REF_PWM = (AAmplitude/5)*100;
      PACE_CHARGE_CTRL = true;
      %Discharge C21
      PACE_GND_CTRL = true;
      VENT_PACE_CTRL = false;
      Z_ATR_CTRL = false;
      Z_VENT_CTRL = false;
      ATR_PACE_CTRL = false;
      VENT_GND_CTRL = false;
      ATR_GND_CTRL = true;
      state = 1;
      prev_state = 2;
    state Discharge_C22_ATR_AOO
      entry:
      %Discharge C22
      PACE_CHARGE_CTRL = false;
      PACE_GND_CTRL = true;
      VENT_PACE_CTRL = false;
      ATR_GND_CTRL = false;
      Z_ATR_CTRL = false;
      Z_VENT_CTRL = false;
      VENT_GND_CTRL = false;
      ATR_PACE_CTRL = true;
      state = 2;
      prev_state = 1;
    AOO.Charge_C22_AOO -> AOO.Discharge_C22_ATR_AOO [order 2] : [after(LRI,msec)]
    AOO.Discharge_C22_ATR_AOO -> AOO.Charge_C22_AOO : after(AtrWidth,msec)
  state AOOR [group]
    state Charge_C22_AOO
      entry:
      %Charge C22
      ATR_PACE_CTRL = false;
      VENT_PACE_CTRL = false;
      PACING_REF_PWM = (AAmplitude/5)*100;
      PACE_CHARGE_CTRL = true;
      %Discharge C21
      PACE_GND_CTRL = true;
      VENT_PACE_CTRL = false;
      Z_ATR_CTRL = false;
      Z_VENT_CTRL = false;
      ATR_PACE_CTRL = false;
      VENT_GND_CTRL = false;
      ATR_GND_CTRL = true;
      state = 1;
      prev_state = 2;
    state Discharge_C22_ATR_AOO
      entry:
      %Discharge C22
      PACE_CHARGE_CTRL = false;
      PACE_GND_CTRL = true;
      VENT_PACE_CTRL = false;
      ATR_GND_CTRL = false;
      Z_ATR_CTRL = false;
      Z_VENT_CTRL = false;
      VENT_GND_CTRL = false;
      ATR_PACE_CTRL = true;
      state = 2;
      prev_state = 1;
    AOOR.Charge_C22_AOO -> AOOR.Discharge_C22_ATR_AOO : [after(interval,msec)]
    AOOR.Discharge_C22_ATR_AOO -> AOOR.Charge_C22_AOO : after(AtrWidth,msec)
  state AAI [group]
    state Wait_AAI %(Refractory Period)
      entry:
      ATR_CMP_REF_PWM = (AtrSensitivity/5)*100;
      FRONTEND_CTRL = false;
      %Discharge C21 and Charge C22
      PACE_GND_CTRL = true;
      VENT_PACE_CTRL = false;
      Z_ATR_CTRL = false;
      Z_VENT_CTRL = false;
      ATR_PACE_CTRL = false;
      VENT_GND_CTRL = false;
      ATR_GND_CTRL = true;
      PACING_REF_PWM = (AAmplitude/5)*100;
      PACE_CHARGE_CTRL = true;
      state = 1;
    state Sensing_Charge_C22_AAI %(Alert Period)
      entry:
      %Sensing turns on
      FRONTEND_CTRL = true;
      %Charge C22
      ATR_PACE_CTRL = false;
      VENT_PACE_CTRL = false;
      PACING_REF_PWM = (AAmplitude/5)*100;
      PACE_CHARGE_CTRL = true;
      state = 2;
      prev_state = 1;
    state Discharge_C22_ATR_AAI %(Pacing)
      entry:
      %Discharge C22, Sensing turns off
      FRONTEND_CTRL = false;
      PACE_CHARGE_CTRL = false;
      PACE_GND_CTRL = true;
      VENT_PACE_CTRL = false;
      ATR_GND_CTRL = false;
      Z_ATR_CTRL = false;
      Z_VENT_CTRL = false;
      VENT_GND_CTRL = false;
      ATR_PACE_CTRL = true;
      state =3;
      prev_state = 2;
    AAI.Wait_AAI %(Refractory Period) -> AAI.Sensing_Charge_C22_AAI %(Alert Period) [order 2] : [after(ARP, msec)]
    AAI.Sensing_Charge_C22_AAI %(Alert Period) -> AAI.Wait_AAI %(Refractory Period) [order 1] : [ATR_CMP_DETECT == true]{natural = true}
    AAI.Sensing_Charge_C22_AAI %(Alert Period) -> AAI.Discharge_C22_ATR_AAI %(Pacing) [order 2] : [after(LRI-ARP-AtrWidth,msec) & ATR_CMP_DETECT == false & natural == false]
    AAI.Sensing_Charge_C22_AAI %(Alert Period) -> AAI.Discharge_C22_ATR_AAI %(Pacing) [order 3] : [after(LRI-ARP,msec) & ATR_CMP_DETECT == false & natural == true]{natural = false}
    AAI.Discharge_C22_ATR_AAI %(Pacing) -> AAI.Wait_AAI %(Refractory Period) : [after(AtrWidth,msec)]
  state AAIR [group]
    state Wait_AAI %(Refractory Period)
      entry:
      ATR_CMP_REF_PWM = (AtrSensitivity/5)*100;
      FRONTEND_CTRL = false;
      %Discharge C21 and Charge C22
      PACE_GND_CTRL = true;
      VENT_PACE_CTRL = false;
      Z_ATR_CTRL = false;
      Z_VENT_CTRL = false;
      ATR_PACE_CTRL = false;
      VENT_GND_CTRL = false;
      ATR_GND_CTRL = true;
      PACING_REF_PWM = (AAmplitude/5)*100;
      PACE_CHARGE_CTRL = true;
      state = 1;
    state Sensing_Charge_C22_AAI %(Alert Period)
      entry:
      %Sensing turns on
      FRONTEND_CTRL = true;
      %Charge C22
      ATR_PACE_CTRL = false;
      VENT_PACE_CTRL = false;
      PACING_REF_PWM = (AAmplitude/5)*100;
      PACE_CHARGE_CTRL = true;
      state = 2;
      prev_state = 1;
    state Discharge_C22_ATR_AAI %(Pacing)
      entry:
      %Discharge C22, Sensing turns off
      FRONTEND_CTRL = false;
      PACE_CHARGE_CTRL = false;
      PACE_GND_CTRL = true;
      VENT_PACE_CTRL = false;
      ATR_GND_CTRL = false;
      Z_ATR_CTRL = false;
      Z_VENT_CTRL = false;
      VENT_GND_CTRL = false;
      ATR_PACE_CTRL = true;
      state =3;
      prev_state = 2;
    AAIR.Sensing_Charge_C22_AAI %(Alert Period) -> AAIR.Wait_AAI %(Refractory Period) [order 1] : [ATR_CMP_DETECT == true]{natural = true}
    AAIR.Wait_AAI %(Refractory Period) -> AAIR.Sensing_Charge_C22_AAI %(Alert Period) : [after(ARP, msec)]
    AAIR.Sensing_Charge_C22_AAI %(Alert Period) -> AAIR.Discharge_C22_ATR_AAI %(Pacing) [order 3] : [after(interval-ARP,msec) & ATR_CMP_DETECT == false & natural == true]{natural = false}
    AAIR.Sensing_Charge_C22_AAI %(Alert Period) -> AAIR.Discharge_C22_ATR_AAI %(Pacing) [order 2] : [after(interval-ARP-AtrWidth,msec) & ATR_CMP_DETECT == false & natural == false]
    AAIR.Discharge_C22_ATR_AAI %(Pacing) -> AAIR.Wait_AAI %(Refractory Period) : [after(AtrWidth,msec)]
  Mode_Selector -> VOOR.Charge_C22_VOO [order 5] : [mode == 5]
  Mode_Selector -> VOO.Charge_C22_VOO [order 1] : [mode == 1]
  VOO.Charge_C22_VOO -> Mode_Selector [order 1] : [mode == 0]
  Mode_Selector -> VVIR.Wait_VVI %(Refractory Period) [order 6] : [mode == 6]
  Mode_Selector -> VVI.Wait_VVI %(Refractory Period) [order 2] : [mode == 2]
  VVI.Wait_VVI %(Refractory Period) -> Mode_Selector [order 1] : [mode == 0]
  (default) -> Mode_Selector
  Mode_Selector -> AOOR.Charge_C22_AOO [order 7] : [mode == 7]
  Mode_Selector -> AOO.Charge_C22_AOO [order 3] : [mode == 3]
  AOO.Charge_C22_AOO -> Mode_Selector [order 1] : [mode == 0]
  Mode_Selector -> AAIR.Wait_AAI %(Refractory Period) [order 8] : [mode == 8]
  AAI.Wait_AAI %(Refractory Period) -> Mode_Selector [order 1] : [mode == 0]
  Mode_Selector -> AAI.Wait_AAI %(Refractory Period) [order 4] : [mode == 4]
  data: ATR_PACE_CTRL output boolean; VENT_PACE_CTRL output boolean; PACING_REF_PWM output double; PACE_CHARGE_CTRL output boolean; PACE_GND_CTRL output boolean; ATR_GND_CTRL output boolean; Z_ATR_CTRL output boolean; Z_VENT_CTRL output boolean; VENT_GND_CTRL output boolean; FRONTEND_CTRL output boolean; VENT_CMP_REF_PWM output double; VENT_CMP_DETECT input boolean; VentWidth input int16; LRL input double; VRP input double [150..500]; ARP input double [150..500]; ATR_CMP_DETECT input boolean; ATR_CMP_REF_PWM output double; mode input int16; VAmplitude input double; AAmplitude input double; state output int16; natural local boolean; prev_state output int16; AtrWidth input int16; VentSensitivity input double; AtrSensitivity input double; LRI local double; AdaptiveRate input double; interval local

== stateflow chart simulink_group46/Test Sequence ==
  state Scenario_1
    state Creating_constant_parameters
      LRL = 60;
      width=5;
      pulse_period=1;
      VAmplitude=4;
      AAmplitude=4;
      VRP=150;
      ARP=150;
      Activity Level=1;
      Mode=1;
      state No_Natural_Heartbeat
        VENT_CMP_DETECT=0;
        settings: description=et = elapsed time
      state Natural_Heartbeat
        VENT_CMP_DETECT=1;
      (default) -> No_Natural_Heartbeat
      No_Natural_Heartbeat -> Natural_Heartbeat : [
          | et>2
          | ]
      Natural_Heartbeat -> No_Natural_Heartbeat : [
          | et>0.005
          | ]
    state step_2
    (default) -> Creating_constant_parameters
    Creating_constant_parameters -> Scenario_1.step_2
  state Scenario_2
    state Creating_Constant_Parameters
      URL=120;
      width=5;
      pulse_period=1;
      VAmplitude=4;
      AAmplitude=4;
      VRP=150;
      ARP=150;
      Activity Level=1;
      Mode=1;
      VENT_CMP_DETECT=0;
      settings: description=How activity level changes over time
      state CONST_ACTIVITY_LEVEL
        Activity Level=3;
      state SINE_ACTIVITY_LEVEL
        Activity Level = 3+30*sin(t*2*pi/30);
        settings: description=Use sine wave to see how activity level changes
      (default) -> CONST_ACTIVITY_LEVEL
      CONST_ACTIVITY_LEVEL -> SINE_ACTIVITY_LEVEL : [
          | et>10
          | ]
      SINE_ACTIVITY_LEVEL -> CONST_ACTIVITY_LEVEL : [
          | Activity Level < 3
          | ]
    state step_2
    (default) -> Creating_Constant_Parameters
    Creating_Constant_Parameters -> Scenario_2.step_2
  (default) -> Scenario_1 [order 1] : [Active_Scenario_Index == 1]
  (default) -> Scenario_2 [order 2] : {assert(Active_Scenario_Index == 2,'The value of Scenario Parameter ''Active_Scenario_Index'' is not valid. Use the index of the scenario to specify it.')}
  data: Active_Scenario_Index parameter =1

== stateflow chart simulink_group46/INPUTS/Obtain Desired ==
  state below
    entry:
    desired = LRL;
    comparator="below";
  state start
    entry:
    comparator = "";
  state within
    entry:
    desired = 10*sqrt(resp_factor*sqrt(threshold)*(level-threshold)) + LRL;
    comparator="within";
  state above
    entry:
    desired = MSR;
    comparator="above";
  (default) -> start
  start -> below [order 1] : [level <= threshold]
  start -> within [order 2] : [level > threshold & level < MSR]
  start -> above [order 3] : [level >= threshold]
  data: desired output double; comparator output string; threshold input double; resp_factor input double; level input double; MSR input double; LRL input double

== stateflow chart simulink_group46/INPUTS/Obtain New Rate ==
  state Adjust_Down
    entry:
    slope = (MSR - LRL)/RecoveryTime;
    NewRate = current - slope/1000;
    adjust="down";
  state Selector
    entry:
    adjust = "";
    current = CurrentRate;
    if (current == 0)
    current = LRL;
    end
  state Adjust_Up
    entry:
    slope = (MSR - LRL)/ReactionTime;
    NewRate = current + slope/1000;
    adjust="up";
  state Hold
    entry:
    NewRate = current;
    adjust="hold";
  Selector -> Adjust_Down [order 1] : [desired > CurrentRate]
  (default) -> Selector
  Selector -> Adjust_Up [order 2] : [desired < CurrentRate]
  Selector -> Hold [order 3] : [desired == CurrentRate]
  data: desired input double; NewRate output double; CurrentRate input double; ReactionTime input double; RecoveryTime input double; MSR input double; LRL input double; adjust output string; current local double; slope local double

== stateflow chart simulink_group46/INPUTS/COM_IN ==
  state SET_PARAM
    entry:
    update = true;
    VRP = typecast(Rx(3:10),'double');
    VentWidth = typecast(Rx(11:12),'int16');
    URL = typecast(Rx(13:20),'double');
    LRL = typecast(Rx(21:28),'double');
    ARP = typecast(Rx(29:36),'double');
    mode = typecast(Rx(37:38),'int16');
    VAmplitude = typecast(Rx(39:46),'double');
    AAmplitude = typecast(Rx(47:54),'double');
    RecoveryTime = typecast(Rx(55:62),'double');
    ResponseFactor = typecast(Rx(63:70),'double');
    ReactionTime = typecast(Rx(71:78),'double');
    ActivityThreshold = typecast(Rx(79:86),'double');
    AtrWidth = typecast(Rx(87:88),'int16');
    MSR = typecast(Rx(89:96),'double');
    VentSensitivity = typecast(Rx(97:104),'double');
    AtrSensitivity = typecast(Rx(105:112),'double');
  state INITIAL
    entry:
    VentWidth = 1;
    AtrWidth = 1;
    URL = 120;
    LRL = 60;
    VRP = 320;
    ARP = 250;
    mode = 0;
    VAmplitude = 4;
    AAmplitude = 4;
    ReactionTime = 30;
    ResponseFactor = 8;
    RecoveryTime = 300;
    ActivityThreshold = 4;
    MSR = 120;
    VentSensitivity = 3.5;
    AtrSensitivity = 3.5;
  state SEND_ECG
    entry:
    type = 0;
    send_params();
  state STANDBY
  state ECHO_PARAM
    entry:
    type = 1;
    send_params();
  (default) -> INITIAL
  SET_PARAM -> STANDBY
  (junction 18) -> SET_PARAM [order 3] : [Rx(2) == hex2dec('22')]
  (junction 14) -> STANDBY [order 2]
  STANDBY -> (junction 14) : [status == 0]{update = false;}
  (junction 14) -> (junction 18) [order 1] : [Rx(1) == hex2dec('16')]
  (junction 18) -> SEND_ECG [order 2] : [Rx(2) == hex2dec('44')]
  INITIAL -> STANDBY
  (junction 18) -> ECHO_PARAM [order 1] : [Rx(2) == hex2dec('33')]
  SEND_ECG -> STANDBY
  ECHO_PARAM -> STANDBY
  data: Rx input uint8; status input uint8; VentWidth output int16; mode output int16; VRP output double; VAmplitude output double; URL output double; LRL output double; ARP output double; AAmplitude output double; RecoveryTime output double; ResponseFactor output double; ReactionTime output double; ActivityThreshold output double; AtrWidth output int16; MSR output double; VentSensitivity output double; AtrSensitivity output double; update output boolean; type output int8
